simulink model "CalcSpinSpeednDir"  (R2020b)
settings: Solver=FixedStepDiscrete  StartTime=0.0  StopTime=100  FixedStep=1  RelTol=1e-3
values from neighbouring files (symbols this model uses):
  p = 4.0    [CalcSpeednDir.sldd]
libraries: simulink x1
settings Model: DataDictionary=CalcSpeednDir.sldd  Creator=unix  LastModifiedBy=unix
settings SolverCC: AutoInsertRateTranBlk=on
settings DataIOCC: SaveOutput=off  SaveTime=off
settings OptimizationCC: DefaultParameterBehavior=Inlined  EnhancedBackFolding=on  PassReuseOutputArgsAs=Individual arguments  ZeroExternalMemoryAtStartup=off  ZeroInternalMemoryAtStartup=off  OptimizeBlockOrder=speed  DifferentSizesBufferReuse=on  OptimizationCustomize=off  EfficientTunableParamExpr=on
settings DebuggingCC: SignalInfNanChecking=warning  SignalRangeChecking=warning  CheckMatrixSingularityMsg=warning  IntegerOverflowMsg=error  ParameterOverflowMsg=warning  ParameterUnderflowMsg=warning  ParameterPrecisionLossMsg=none  ParameterTunabilityLossMsg=error  UnderSpecifiedDataTypeMsg=warning  IntegerSaturationMsg=error
settings SFSimCC: MATLABDynamicMemAlloc=off
settings RTWCC: Description=Embedded Coder  SystemTargetFile=ert.tlc  GenCodeOnly=on  TemplateMakefile=ert_default_tmf  GenerateReport=on  IncludeHyperlinkInReport=on  LaunchReport=on  GenerateTraceInfo=on  GenerateTraceReport=on  GenerateTraceReportSl=on  GenerateTraceReportSf=on  GenerateTraceReportEml=on
settings CodeAppCC: ForceParamTrailComments=on  IgnoreCustomStorageClasses=off  OperatorAnnotations=on  SimulinkDataObjDesc=on  SFDataObjDesc=on  InsertBlockDesc=on
settings ERTTargetCC: TargetLangStandard=C99 (ISO)  GenerateSampleERTMain=on  GenerateASAP2=on  InlinedParameterPlacement=NonHierarchical  ERTCustomFileTemplate=example_file_process.tlc

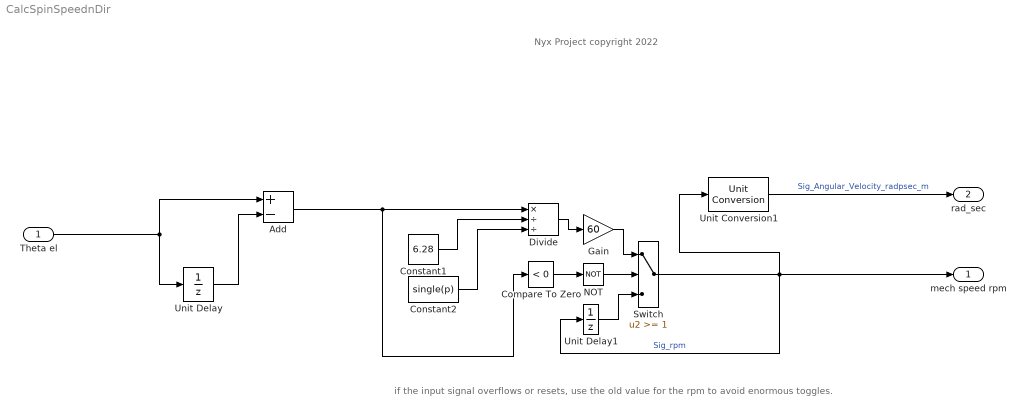
== system CalcSpinSpeednDir ==
  note: Nyx Project copyright 2022
  note: if the input signal overflows or resets, use the old value for the rpm to avoid enormous toggles.
  Theta el : Inport  OutDataTypeStr=single
  Add : Sum  Inputs=+-
  Compare To Zero : simulink/Logic and Bit Operations/Compare To Zero  relop=<  OutDataTypeStr=boolean
  Constant1 : Constant  Value=6.28  OutDataTypeStr=single
  Constant2 : Constant  Value=single(p)  OutDataTypeStr=single
  Divide : Product  Inputs=*//  OutDataTypeStr=int32
  Gain : Gain  Gain=60
  NOT : Logic  Operator=NOT  IconShape=distinctive  AllPortsSameDT=off  OutDataTypeStr=boolean
  Switch : Switch  Threshold=1
  Unit Conversion1 : UnitConversion  OutputType=Inherit: Inherit via back propagation
  Unit Delay : UnitDelay  SampleTime=-1  HasFrameUpgradeWarning=on
  Unit Delay1 : UnitDelay  SampleTime=-1  HasFrameUpgradeWarning=on
  mech speed rpm : Outport
  rad_sec : Outport  Port=2  OutDataTypeStr=single  Unit=rad/sec  PortDimensions=1
  wires:
  Divide/1 -> Gain/1
  Unit Conversion1/1 -> rad_sec/1  "Sig_Angular_Velocity_radpsec_m"
  Constant2/1 -> Divide/3
  Unit Delay/1 -> Add/2
  Theta el/1 -> Add/1, Unit Delay/1
  Constant1/1 -> Divide/2
  Add/1 -> Divide/1, Compare To Zero/1
  Unit Delay1/1 -> Switch/3
  Switch/1 -> Unit Conversion1/1, Unit Delay1/1, mech speed rpm/1  "Sig_rpm"
  Compare To Zero/1 -> NOT/1
  NOT/1 -> Switch/2
  Gain/1 -> Switch/1
